simulink model "sim_model"  (R2021b)
settings: Solver=VariableStepAuto  StartTime=0.0  StopTime=t_final  RelTol=1e-3
values from neighbouring files (symbols this model uses):
  A = [0 0 0 0 0 0 1 -0.898373961449 0 3.85017418861 0 5.13356542587 ... (36 elements, 6x6)]    [AB.mat]    (also in lqr_stuff.m = double(A))
  B = [0 2.13949513435 0 -9.1692647934 0 -12.2256860733]    [AB.mat]    (also in lqr_stuff.m = double(B))
  C = eye(6)    [lqr_stuff.m]
  D = zeros(6,1)    [lqr_stuff.m]
  K_r = 1/(D+C*inv(-A+B*K_lqr)*B)    [lqr_stuff.m]
  Va_max = 24    [lqr_stuff.m]
  x0 = [0; 0; -15/180*pi; 0; -15/180*pi; 0;]    [lqr_stuff.m]
undefined symbols (not defined in the file or in its folder): K_lqr
settings Model: Creator=sacka  LastModifiedBy=sacka

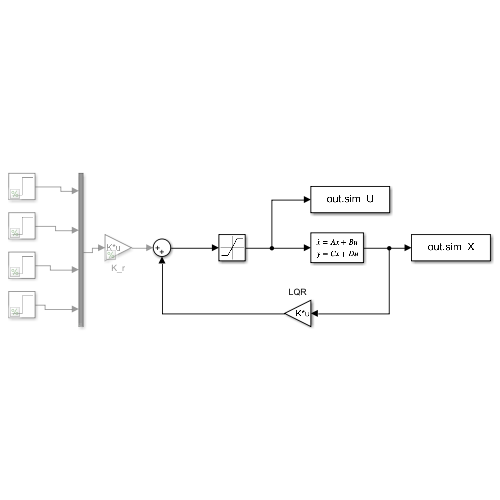
[thumbnail: Simulink's stored preview of the top-level diagram]
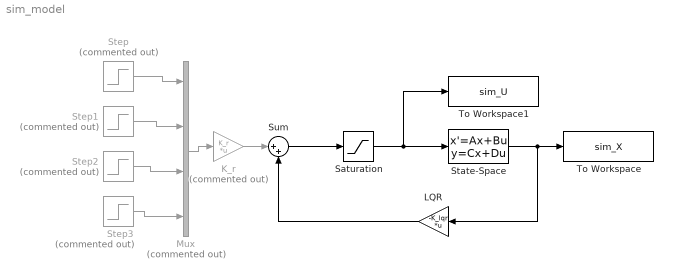
== system sim_model ==
  K_r : Gain  Commented=on  Gain=K_r  Multiplication=Matrix(K*u)
  LQR : Gain  Gain=-K_lqr  Multiplication=Matrix(K*u)
  Mux : Mux  Commented=on
  Saturation : Saturate  UpperLimit=Va_max  LowerLimit=-Va_max
  State-Space : StateSpace  A=A  B=B  C=C  D=D  InitialCondition=x0  ParameterTunability=Unconstrained
  Step : Step  Commented=on  Time=0  Before=0.1  After=0.1  SampleTime=0  ZeroCross=off
  Step1 : Step  Commented=on  Time=0  After=0  SampleTime=0  ZeroCross=off
  Step2 : Step  Commented=on  Time=0  After=0  SampleTime=0  ZeroCross=off
  Step3 : Step  Commented=on  Time=0  After=0  SampleTime=0  ZeroCross=off
  Sum : Sum  Inputs=|++
  To Workspace : ToWorkspace  VariableName=sim_X  SaveFormat=Structure With Time  SampleTime=-1
  To Workspace1 : ToWorkspace  VariableName=sim_U  SaveFormat=Structure With Time  SampleTime=-1
  wires:
  State-Space/1 -> LQR/1, To Workspace/1
  Step/1 -> Mux/1
  Step1/1 -> Mux/2
  Step2/1 -> Mux/3
  Step3/1 -> Mux/4
  Sum/1 -> Saturation/1
  Saturation/1 -> To Workspace1/1, State-Space/1
  Mux/1 -> K_r/1
  K_r/1 -> Sum/1
  LQR/1 -> Sum/2
